simulink model "feedback_linearization_sim_18"  (R2021b)
settings: Solver=VariableStepAuto  StartTime=0.0  StopTime=1000  RelTol=1e-3
undefined symbols (not defined in the file): sim_output_sample_time, sim_r
libraries: simulink x1
settings Model: Creator=alefr  LastModifiedBy=alefr
settings SolverCC: AlgebraicLoopSolver=TrustRegion
settings DataIOCC: ReturnWorkspaceOutputs=off
settings DebuggingCC: ArithmeticOperatorsInVariantConditions=warning
settings SFSimCC: CustomCodeUndefinedFunction=UseInterfaceOnly

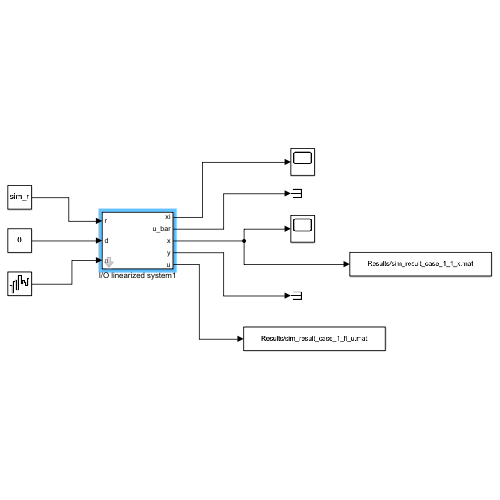
[thumbnail: Simulink's stored preview of the top-level diagram]
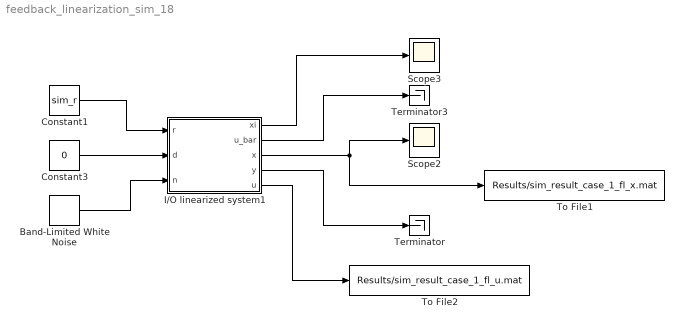
== system feedback_linearization_sim_18 ==
  Band-Limited White Noise : simulink/Sources/Band-Limited White Noise  Cov=0.00001  Ts=0.1  seed=[23341]
  Constant1 : Constant  Value=sim_r
  Constant3 : Constant  Value=0
  I/O linearized system1 : Subsystem  mask{init_state_param=[8;8], integrator_gain_param=0.01}
      mask prompts: init_state_param "Initial state"; integrator_gain_param "Integrator gain"
  Scope2 : Scope
  Scope3 : Scope
  Terminator : Terminator
  Terminator3 : Terminator
  To File1 : ToFile  Filename=Results/sim_result_case_1_fl_x.mat  MatrixName=sim_result_case_1_fl_x  SaveFormat=Timeseries  SampleTime=sim_output_sample_time
  To File2 : ToFile  Filename=Results/sim_result_case_1_fl_u.mat  MatrixName=sim_result_case_1_fl_u  SaveFormat=Timeseries  SampleTime=sim_output_sample_time
  wires:
  I/O linearized system1/4(y) -> Terminator/1
  I/O linearized system1/3(x) -> To File1/1, Scope2/1
  I/O linearized system1/2(u_bar) -> Terminator3/1
  I/O linearized system1/1(xi) -> Scope3/1
  Constant1/1 -> I/O linearized system1/1(r)
  Band-Limited White Noise/1 -> I/O linearized system1/3(n)
  Constant3/1 -> I/O linearized system1/2(d)
  I/O linearized system1/5(u) -> To File2/1

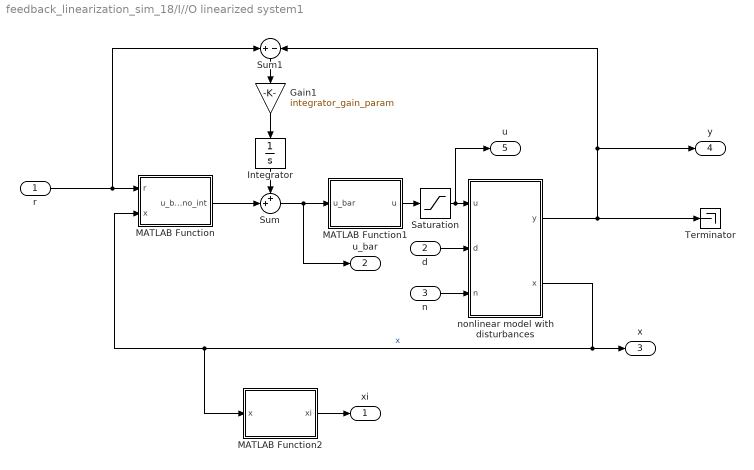
== system feedback_linearization_sim_18/I//O linearized system1 ==
  r : Inport
  d : Inport  Port=2
  n : Inport  Port=3
  Gain1 : Gain  Gain=integrator_gain_param
  Integrator : Integrator
  MATLAB Function : MATLAB Function  TreatAsAtomicUnit=on
  MATLAB Function1 : MATLAB Function  TreatAsAtomicUnit=on
  MATLAB Function2 : MATLAB Function  TreatAsAtomicUnit=on
  Saturation : Saturate  UpperLimit=10  LowerLimit=0
  Sum : Sum  Inputs=++|
  Sum1 : Sum  Inputs=+-
  Terminator : Terminator
  nonlinear model with disturbances : Subsystem
  xi : Outport
  u_bar : Outport  Port=2
  x : Outport  Port=3
  y : Outport  Port=4
  u : Outport  Port=5
  wires:
  n/1 -> nonlinear model with disturbances/3(n)
  d/1 -> nonlinear model with disturbances/2(d)
  nonlinear model with disturbances/2(x) -> x/1, MATLAB Function/2(x), MATLAB Function2/1(x)  "x"
  r/1 -> Sum1/1, MATLAB Function/1(r)
  MATLAB Function2/1(xi) -> xi/1
  Sum/1 -> u_bar/1, MATLAB Function1/1(u_bar)
  MATLAB Function/1(u_bar_no_int) -> Sum/2
  nonlinear model with disturbances/1(y) -> Sum1/2, y/1, Terminator/1
  Sum1/1 -> Gain1/1
  Gain1/1 -> Integrator/1
  Integrator/1 -> Sum/1
  MATLAB Function1/1(u) -> Saturation/1
  Saturation/1 -> u/1, nonlinear model with disturbances/1(u)

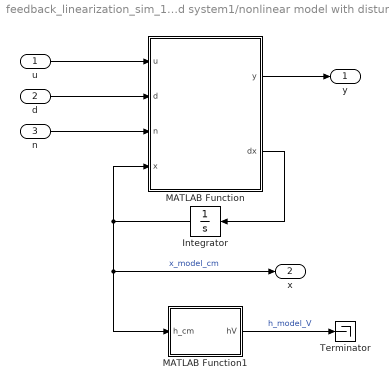
== system feedback_linearization_sim_18/I//O linearized system1/nonlinear model with disturbances ==
  u : Inport
  d : Inport  Port=2
  n : Inport  Port=3
  Integrator : Integrator  InitialCondition=init_state_param
  MATLAB Function : MATLAB Function  TreatAsAtomicUnit=on
  MATLAB Function1 : MATLAB Function  TreatAsAtomicUnit=on
  Terminator : Terminator
  y : Outport
  x : Outport  Port=2
  wires:
  u/1 -> MATLAB Function/1(u)
  Integrator/1 -> x/1, MATLAB Function1/1(h_cm), MATLAB Function/4(x)  "x_model_cm"
  MATLAB Function/2(dx) -> Integrator/1
  d/1 -> MATLAB Function/2(d)
  MATLAB Function1/1(hV) -> Terminator/1  "h_model_V"
  n/1 -> MATLAB Function/3(n)
  MATLAB Function/1(y) -> y/1

== matlab function feedback_linearization_sim_18/I//O linearized system1/MATLAB Function ==
  data: r input; u_bar_no_int output; x input
function u_bar_no_int = k(r,x)

x1 = x(1);
x2 = x(2);

u_bar_no_int = sqrt(x1.*1.962e+3+6.2784e+3).*(r.*(3.0./8.0e+2)-x2.*2.796158531714332e-3+1.0./sqrt(x2.*1.962e+3+6.2784e+3).*(sqrt(x1.*1.962e+3+6.2784e+3).*5.151515151515152e-3-sqrt(x2.*1.962e+3+6.2784e+3).*5.151515151515152e-3).*3.768204915830296-sqrt(x1.*1.962e+3+6.2784e+3).*4.801484347388247e-4+sqrt(x2.*1.962e+3+6.2784e+3).*4.801484347388247e-4+2.559221365943785e-2).*8.757485523509194;

end

== matlab function feedback_linearization_sim_18/I//O linearized system1/MATLAB Function1 ==
  data: u_bar input; u output
function u = pm1(u_bar)

u = u_bar.*3.277899884284337e-1-u_bar.^2.*9.88758313621772e-3+u_bar.^3.*1.567756031883916e-4-2.914041336753123;

end

== matlab function feedback_linearization_sim_18/I//O linearized system1/MATLAB Function2 ==
  data: x input; xi output
function xi = T(x)

x1 = x(1);
x2 = x(2);

xi = [x2.*7.456422751238219e-1-1.648066384406454;sqrt(x1.*1.962e+3+6.2784e+3).*3.841187477910597e-3-sqrt(x2.*1.962e+3+6.2784e+3).*3.841187477910597e-3];

end

== matlab function feedback_linearization_sim_18/I//O linearized system1/nonlinear model with disturbances/MATLAB Function ==
  data: y output; u input; dx output; d input; n input; x input
function [y,dx] = nonlinear_model(u,d,n,x)

x1 = x(1);
x2 = x(2);

y = x2.*7.456422751238219e-1 + n -1.648066384406454;

dx = [+u.*2.81859116712929e-1-(d.*sqrt(x1.*1.962e+3+6.2784e+3))./3.3e+1-sqrt(x1.*1.962e+3+6.2784e+3).*5.151515151515152e-3-u.^2.*2.476601319356692e-2+u.^3.*8.808489605974731e-4+3.751072019731428e-1;sqrt(x1.*1.962e+3+6.2784e+3).*5.151515151515152e-3-sqrt(x2.*1.962e+3+6.2784e+3).*5.151515151515152e-3];

end

== matlab function feedback_linearization_sim_18/I//O linearized system1/nonlinear model with disturbances/MATLAB Function1 ==
  data: h_cm input; hV output
function hV = g(h_cm)

hV = h_cm*7.456422751238219e-1 - 1.648066384406454;
